simulink model "gm_rmsNormalization"  (R2025a)
settings: Solver=FixedStepDiscrete  StartTime=0.0  StopTime=simStopTime  FixedStep=1  RelTol=1e-3
libraries: simulink x23
(part 1 of 3)
settings Model: Creator=yang  LastModifiedBy=yang
settings OptimizationCC: BlockReduction=off  ConditionallyExecuteInputs=off  DefaultParameterBehavior=Inlined
settings DebuggingCC: InheritedTsInSrcMsg=none  SingleTaskRateTransMsg=error

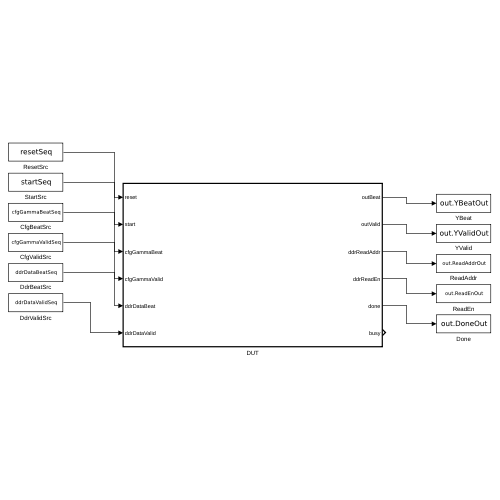
[thumbnail: Simulink's stored preview of the top-level diagram]
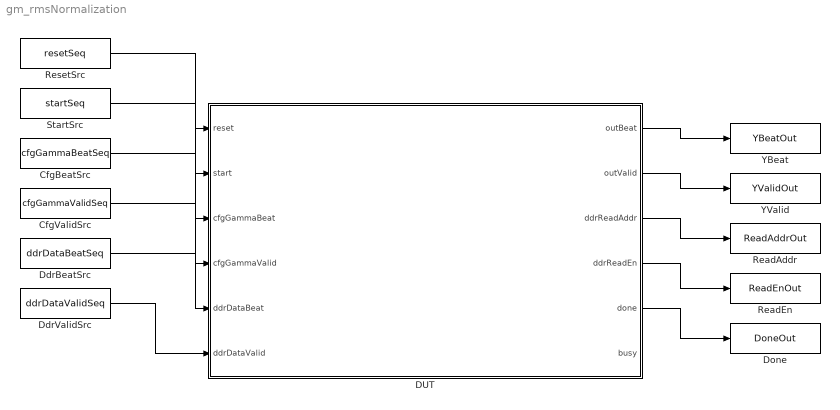
== system gm_rmsNormalization ==
  CfgBeatSrc : FromWorkspace  VariableName=cfgGammaBeatSeq
  CfgValidSrc : FromWorkspace  VariableName=cfgGammaValidSeq
  DUT : Subsystem  TreatAsAtomicUnit=on
  DdrBeatSrc : FromWorkspace  VariableName=ddrDataBeatSeq
  DdrValidSrc : FromWorkspace  VariableName=ddrDataValidSeq
  Done : ToWorkspace  VariableName=DoneOut  SampleTime=-1
  ReadAddr : ToWorkspace  VariableName=ReadAddrOut  SampleTime=-1
  ReadEn : ToWorkspace  VariableName=ReadEnOut  SampleTime=-1
  ResetSrc : FromWorkspace  VariableName=resetSeq
  StartSrc : FromWorkspace  VariableName=startSeq
  YBeat : ToWorkspace  VariableName=YBeatOut  SampleTime=-1
  YValid : ToWorkspace  VariableName=YValidOut  SampleTime=-1
  wires:
  DUT/5(done) -> Done/1
  DUT/4(ddrReadEn) -> ReadEn/1
  DUT/3(ddrReadAddr) -> ReadAddr/1
  DUT/2(outValid) -> YValid/1
  DUT/1(outBeat) -> YBeat/1
  DdrValidSrc/1 -> DUT/6(ddrDataValid)
  DdrBeatSrc/1 -> DUT/5(ddrDataBeat)
  CfgValidSrc/1 -> DUT/4(cfgGammaValid)
  CfgBeatSrc/1 -> DUT/3(cfgGammaBeat)
  StartSrc/1 -> DUT/2(start)
  ResetSrc/1 -> DUT/1(reset)

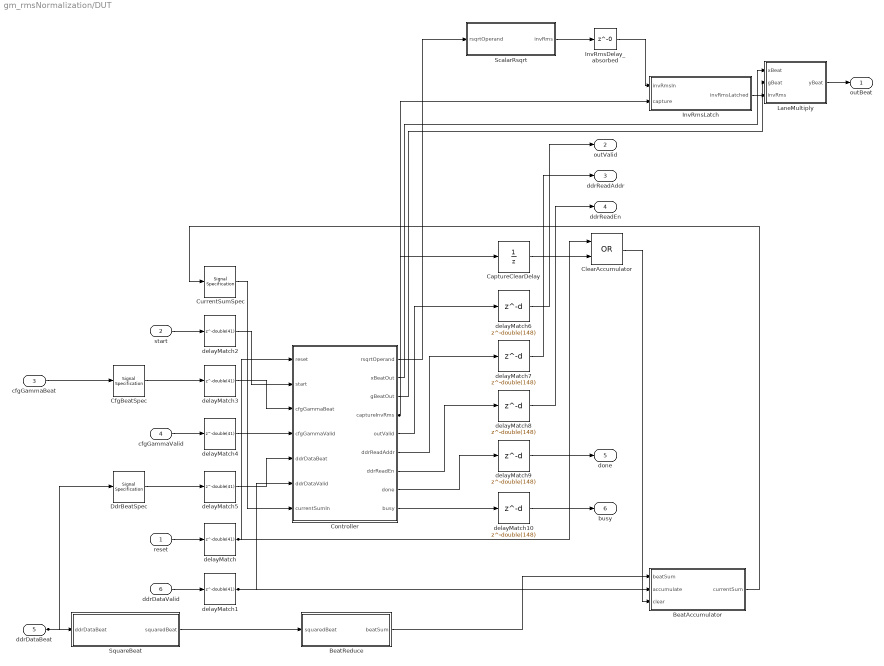
== system gm_rmsNormalization/DUT ==
  reset : Inport  OutDataTypeStr=boolean  PortDimensions=1  SampleTime=1
  start : Inport  Port=2  OutDataTypeStr=boolean  PortDimensions=1  SampleTime=1
  cfgGammaBeat : Inport  Port=3  OutDataTypeStr=single  PortDimensions=[8]  SampleTime=1
  cfgGammaValid : Inport  Port=4  OutDataTypeStr=boolean  PortDimensions=1  SampleTime=1
  ddrDataBeat : Inport  Port=5  OutDataTypeStr=single  PortDimensions=[8]  SampleTime=1
  ddrDataValid : Inport  Port=6  OutDataTypeStr=boolean  PortDimensions=1  SampleTime=1
  BeatAccumulator : Subsystem
  BeatReduce : Subsystem
  CaptureClearDelay : UnitDelay  SampleTime=1
  CfgBeatSpec : SignalSpecification  OutDataTypeStr=single  Dimensions=8
  ClearAccumulator : Logic  Operator=OR  AllPortsSameDT=off  OutDataTypeStr=boolean  SampleTime=1
  Controller : Subsystem
  CurrentSumSpec : SignalSpecification  OutDataTypeStr=single  Dimensions=1
  DdrBeatSpec : SignalSpecification  OutDataTypeStr=single  Dimensions=8
  InvRmsDelay_absorbed : Delay  DelayLength=0
  InvRmsLatch : Subsystem
  LaneMultiply : Subsystem
  ScalarRsqrt : Subsystem
  SquareBeat : Subsystem
  delayMatch{,1..5} (6 alike) : Delay  DelayLength=double(41)  InitialCondition=0  SampleTime=1
  delayMatch{6..10} (5 alike) : Delay  DelayLength=double(148)  InitialCondition=0  SampleTime=1
  outBeat : Outport  SampleTime=1
  outValid : Outport  Port=2  SampleTime=1
  ddrReadAddr : Outport  Port=3  SampleTime=1
  ddrReadEn : Outport  Port=4  SampleTime=1
  done : Outport  Port=5  SampleTime=1
  busy : Outport  Port=6  SampleTime=1
  wires:
  LaneMultiply/1(yBeat) -> outBeat/1
  ClearAccumulator/1 -> BeatAccumulator/3(clear)
  InvRmsDelay_absorbed/1 -> InvRmsLatch/1(invRmsIn)
  delayMatch10/1 -> busy/1
  delayMatch9/1 -> done/1
  delayMatch8/1 -> ddrReadEn/1
  InvRmsLatch/1(invRmsLatched) -> LaneMultiply/3(invRms)
  delayMatch7/1 -> ddrReadAddr/1
  CurrentSumSpec/1 -> Controller/7(currentSumIn)
  delayMatch2/1 -> Controller/2(start)
  ScalarRsqrt/1(invRms) -> InvRmsDelay_absorbed/1
  ddrDataValid/1 -> delayMatch1/1
  DdrBeatSpec/1 -> delayMatch5/1
  cfgGammaValid/1 -> delayMatch4/1
  BeatAccumulator/1(currentSum) -> CurrentSumSpec/1
  CfgBeatSpec/1 -> delayMatch3/1
  Controller/4(captureInvRms) -> CaptureClearDelay/1, InvRmsLatch/2(capture)
  SquareBeat/1(squaredBeat) -> BeatReduce/1(squaredBeat)
  start/1 -> delayMatch2/1
  Controller/7(ddrReadEn) -> delayMatch8/1
  reset/1 -> delayMatch/1
  ddrDataBeat/1 -> SquareBeat/1(ddrDataBeat), DdrBeatSpec/1
  delayMatch5/1 -> Controller/5(ddrDataBeat)
  cfgGammaBeat/1 -> CfgBeatSpec/1
  BeatReduce/1(beatSum) -> BeatAccumulator/1(beatSum)
  delayMatch4/1 -> Controller/4(cfgGammaValid)
  delayMatch/1 -> Controller/1(reset), ClearAccumulator/1
  delayMatch3/1 -> Controller/3(cfgGammaBeat)
  delayMatch1/1 -> Controller/6(ddrDataValid), BeatAccumulator/2(accumulate)
  Controller/5(outValid) -> delayMatch6/1
  Controller/1(rsqrtOperand) -> ScalarRsqrt/1(rsqrtOperand)
  Controller/2(xBeatOut) -> LaneMultiply/1(xBeat)
  Controller/3(gBeatOut) -> LaneMultiply/2(gBeat)
  Controller/6(ddrReadAddr) -> delayMatch7/1
  Controller/8(done) -> delayMatch9/1
  Controller/9(busy) -> delayMatch10/1
  CaptureClearDelay/1 -> ClearAccumulator/2
  delayMatch6/1 -> outValid/1

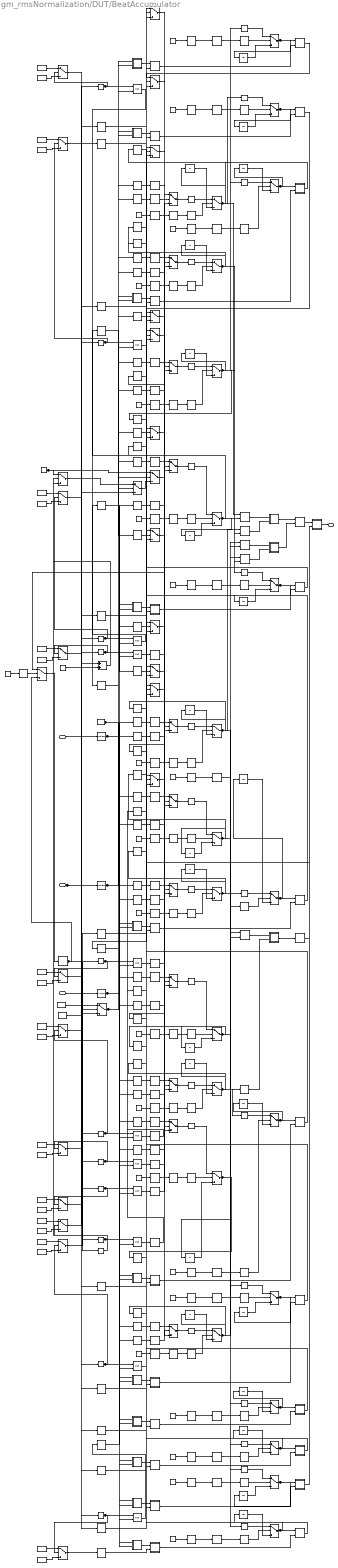
== system gm_rmsNormalization/DUT/BeatAccumulator ==
  beatSum : Inport  OutDataTypeStr=single  PortDimensions=1  SampleTime=1
  accumulate : Inport  Port=2  OutDataTypeStr=boolean  PortDimensions=1  SampleTime=1
  clear : Inport  Port=3  OutDataTypeStr=boolean  PortDimensions=1  SampleTime=1
  AccumulateAdd00 : Subsystem
      mask Display: disp('NFP\nadd');
  AccumulateAdd01 : Subsystem
      mask Display: disp('NFP\nadd');
  AccumulateAdd02 : Subsystem
      mask Display: disp('NFP\nadd');
  AccumulateAdd03 : Subsystem
      mask Display: disp('NFP\nadd');
  AccumulateAdd04 : Subsystem
      mask Display: disp('NFP\nadd');
  AccumulateAdd05 : Subsystem
      mask Display: disp('NFP\nadd');
  AccumulateAdd06 : Subsystem
      mask Display: disp('NFP\nadd');
  AccumulateAdd07 : Subsystem
      mask Display: disp('NFP\nadd');
  AccumulateAdd08 : Subsystem
      mask Display: disp('NFP\nadd');
  AccumulateAdd09 : Subsystem
      mask Display: disp('NFP\nadd');
  AccumulateAdd10 : Subsystem
      mask Display: disp('NFP\nadd');
  AccumulateBool : DataTypeConversion  OutDataTypeStr=boolean
  BankIndexAdd : Sum  OutDataTypeStr=uint8  AccumDataTypeStr=uint8  SampleTime=1
  BankIndexAdvance : Switch  Criteria=u2 ~= 0  Threshold="fi(0,0,1,0,\"hex\",\"0\")"  OutDataTypeStr=uint8  SampleTime=1  SaturateOnIntegerOverflow=off  InputSameDT=off
  BankIndexClear : Switch  Criteria=u2 ~= 0  Threshold="fi(0,0,1,0,\"hex\",\"0\")"  OutDataTypeStr=uint8  SampleTime=1  SaturateOnIntegerOverflow=off  InputSameDT=off
  BankIndexIsLast : simulink/Logic and Bit Operations/Compare To Constant  relop===  const="fi(0,0,8,0,\"hex\",\"0a\")"  OutDataTypeStr=boolean
  BankIndexOne : Constant  OutDataTypeStr=uint8  SampleTime=1
  BankIndexState : Delay  DelayLength=double(1)  InitialCondition=0  SampleTime=1
  BankIndexState_enbsw : Switch  Criteria=u2 ~= 0  Threshold=double(0)  OutDataTypeStr=uint8  SampleTime=1  SaturateOnIntegerOverflow=off  InputSameDT=off
  BankIndexWrap : Switch  Criteria=u2 ~= 0  Threshold="fi(0,0,1,0,\"hex\",\"0\")"  OutDataTypeStr=uint8  SampleTime=1  SaturateOnIntegerOverflow=off  InputSameDT=off
  BankIndexZero : Constant  Value=0  OutDataTypeStr=uint8  SampleTime=1
  BankState00_absorbed : Delay  DelayLength=0
  BankState00_out1bypassMux : Switch  Criteria=u2 ~= 0  Threshold=double(0)  OutDataTypeStr=single  SampleTime=1  SaturateOnIntegerOverflow=off  InputSameDT=off
  BankState01_absorbed : Delay  DelayLength=0
  BankState01_out1bypassMux : Switch  Criteria=u2 ~= 0  Threshold=double(0)  OutDataTypeStr=single  SampleTime=1  SaturateOnIntegerOverflow=off  InputSameDT=off
  BankState02_absorbed : Delay  DelayLength=0
  BankState02_out1bypassMux : Switch  Criteria=u2 ~= 0  Threshold=double(0)  OutDataTypeStr=single  SampleTime=1  SaturateOnIntegerOverflow=off  InputSameDT=off
  BankState03_absorbed : Delay  DelayLength=0
  BankState03_out1bypassMux : Switch  Criteria=u2 ~= 0  Threshold=double(0)  OutDataTypeStr=single  SampleTime=1  SaturateOnIntegerOverflow=off  InputSameDT=off
  BankState04_absorbed : Delay  DelayLength=0
  BankState04_out1bypassMux : Switch  Criteria=u2 ~= 0  Threshold=double(0)  OutDataTypeStr=single  SampleTime=1  SaturateOnIntegerOverflow=off  InputSameDT=off
  BankState05_absorbed : Delay  DelayLength=0
  BankState05_out1bypassMux : Switch  Criteria=u2 ~= 0  Threshold=double(0)  OutDataTypeStr=single  SampleTime=1  SaturateOnIntegerOverflow=off  InputSameDT=off
  BankState06_absorbed : Delay  DelayLength=0
  BankState06_out1bypassMux : Switch  Criteria=u2 ~= 0  Threshold=double(0)  OutDataTypeStr=single  SampleTime=1  SaturateOnIntegerOverflow=off  InputSameDT=off
  BankState07_absorbed : Delay  DelayLength=0
  BankState07_out1bypassMux : Switch  Criteria=u2 ~= 0  Threshold=double(0)  OutDataTypeStr=single  SampleTime=1  SaturateOnIntegerOverflow=off  InputSameDT=off
  BankState08_absorbed : Delay  DelayLength=0
  BankState08_out1bypassMux : Switch  Criteria=u2 ~= 0  Threshold=double(0)  OutDataTypeStr=single  SampleTime=1  SaturateOnIntegerOverflow=off  InputSameDT=off
  BankState09_absorbed : Delay  DelayLength=0
  BankState09_out1bypassMux : Switch  Criteria=u2 ~= 0  Threshold=double(0)  OutDataTypeStr=single  SampleTime=1  SaturateOnIntegerOverflow=off  InputSameDT=off
  BankState10_absorbed : Delay  DelayLength=0
  BankState10_out1bypassMux : Switch  Criteria=u2 ~= 0  Threshold=double(0)  OutDataTypeStr=single  SampleTime=1  SaturateOnIntegerOverflow=off  InputSameDT=off
  BeatSumSingle : DataTypeConversion  OutDataTypeStr=single
  ClearBool : DataTypeConversion  OutDataTypeStr=boolean
  ClearPipe00 : Switch  Criteria=u2 ~= 0  Threshold="fi(0,0,1,0,\"hex\",\"0\")"  OutDataTypeStr=single  SampleTime=1  SaturateOnIntegerOverflow=off  InputSameDT=off
  ClearPipe01 : Switch  Criteria=u2 ~= 0  Threshold="fi(0,0,1,0,\"hex\",\"0\")"  OutDataTypeStr=single  SampleTime=1  SaturateOnIntegerOverflow=off  InputSameDT=off
  ClearPipe02 : Switch  Criteria=u2 ~= 0  Threshold="fi(0,0,1,0,\"hex\",\"0\")"  OutDataTypeStr=single  SampleTime=1  SaturateOnIntegerOverflow=off  InputSameDT=off
  ClearPipe03 : Switch  Criteria=u2 ~= 0  Threshold="fi(0,0,1,0,\"hex\",\"0\")"  OutDataTypeStr=single  SampleTime=1  SaturateOnIntegerOverflow=off  InputSameDT=off
  ClearPipe04 : Switch  Criteria=u2 ~= 0  Threshold="fi(0,0,1,0,\"hex\",\"0\")"  OutDataTypeStr=single  SampleTime=1  SaturateOnIntegerOverflow=off  InputSameDT=off
  ClearPipe05 : Switch  Criteria=u2 ~= 0  Threshold="fi(0,0,1,0,\"hex\",\"0\")"  OutDataTypeStr=single  SampleTime=1  SaturateOnIntegerOverflow=off  InputSameDT=off
  ClearPipe06 : Switch  Criteria=u2 ~= 0  Threshold="fi(0,0,1,0,\"hex\",\"0\")"  OutDataTypeStr=single  SampleTime=1  SaturateOnIntegerOverflow=off  InputSameDT=off
  ClearPipe07 : Switch  Criteria=u2 ~= 0  Threshold="fi(0,0,1,0,\"hex\",\"0\")"  OutDataTypeStr=single  SampleTime=1  SaturateOnIntegerOverflow=off  InputSameDT=off
  ClearPipe08 : Switch  Criteria=u2 ~= 0  Threshold="fi(0,0,1,0,\"hex\",\"0\")"  OutDataTypeStr=single  SampleTime=1  SaturateOnIntegerOverflow=off  InputSameDT=off
  ClearPipe09 : Switch  Criteria=u2 ~= 0  Threshold="fi(0,0,1,0,\"hex\",\"0\")"  OutDataTypeStr=single  SampleTime=1  SaturateOnIntegerOverflow=off  InputSameDT=off
  ClearPipe10 : Switch  Criteria=u2 ~= 0  Threshold="fi(0,0,1,0,\"hex\",\"0\")"  OutDataTypeStr=single  SampleTime=1  SaturateOnIntegerOverflow=off  InputSameDT=off
  FeedbackDelay00_absorbed : Delay  DelayLength=0
  FeedbackDelay00_out1bypassMux : Switch  Criteria=u2 ~= 0  Threshold=double(0)  OutDataTypeStr=single  SampleTime=1  SaturateOnIntegerOverflow=off  InputSameDT=off
  FeedbackDelay01_absorbed : Delay  DelayLength=0
  FeedbackDelay01_out1bypassMux : Switch  Criteria=u2 ~= 0  Threshold=double(0)  OutDataTypeStr=single  SampleTime=1  SaturateOnIntegerOverflow=off  InputSameDT=off
  FeedbackDelay02_absorbed : Delay  DelayLength=0
  FeedbackDelay02_out1bypassMux : Switch  Criteria=u2 ~= 0  Threshold=double(0)  OutDataTypeStr=single  SampleTime=1  SaturateOnIntegerOverflow=off  InputSameDT=off
  FeedbackDelay03_absorbed : Delay  DelayLength=0
  FeedbackDelay03_out1bypassMux : Switch  Criteria=u2 ~= 0  Threshold=double(0)  OutDataTypeStr=single  SampleTime=1  SaturateOnIntegerOverflow=off  InputSameDT=off
  FeedbackDelay04_absorbed : Delay  DelayLength=0
  FeedbackDelay04_out1bypassMux : Switch  Criteria=u2 ~= 0  Threshold=double(0)  OutDataTypeStr=single  SampleTime=1  SaturateOnIntegerOverflow=off  InputSameDT=off
  FeedbackDelay05_absorbed : Delay  DelayLength=0
  FeedbackDelay05_out1bypassMux : Switch  Criteria=u2 ~= 0  Threshold=double(0)  OutDataTypeStr=single  SampleTime=1  SaturateOnIntegerOverflow=off  InputSameDT=off
  FeedbackDelay06_absorbed : Delay  DelayLength=0
  FeedbackDelay06_out1bypassMux : Switch  Criteria=u2 ~= 0  Threshold=double(0)  OutDataTypeStr=single  SampleTime=1  SaturateOnIntegerOverflow=off  InputSameDT=off
  FeedbackDelay07_absorbed : Delay  DelayLength=0
  FeedbackDelay07_out1bypassMux : Switch  Criteria=u2 ~= 0  Threshold=double(0)  OutDataTypeStr=single  SampleTime=1  SaturateOnIntegerOverflow=off  InputSameDT=off
  FeedbackDelay08_absorbed : Delay  DelayLength=0
  FeedbackDelay08_out1bypassMux : Switch  Criteria=u2 ~= 0  Threshold=double(0)  OutDataTypeStr=single  SampleTime=1  SaturateOnIntegerOverflow=off  InputSameDT=off
  FeedbackDelay09_absorbed : Delay  DelayLength=0
  FeedbackDelay09_out1bypassMux : Switch  Criteria=u2 ~= 0  Threshold=double(0)  OutDataTypeStr=single  SampleTime=1  SaturateOnIntegerOverflow=off  InputSameDT=off
  FeedbackDelay10_absorbed : Delay  DelayLength=0
  FeedbackDelay10_out1bypassMux : Switch  Criteria=u2 ~= 0  Threshold=double(0)  OutDataTypeStr=single  SampleTime=1  SaturateOnIntegerOverflow=off  InputSameDT=off
  Gate00 : Subsystem
      mask Display: disp('NFP\nmul');
  Gate001 : Subsystem
      mask Display: disp('NFP\nmul');
  Gate01 : Subsystem
      mask Display: disp('NFP\nmul');
  Gate011 : Subsystem
      mask Display: disp('NFP\nmul');
  Gate02 : Subsystem
      mask Display: disp('NFP\nmul');
  Gate021 : Subsystem
      mask Display: disp('NFP\nmul');
  Gate03 : Subsystem
      mask Display: disp('NFP\nmul');
  Gate031 : Subsystem
      mask Display: disp('NFP\nmul');
  Gate04 : Subsystem
      mask Display: disp('NFP\nmul');
  Gate041 : Subsystem
      mask Display: disp('NFP\nmul');
  Gate05 : Subsystem
      mask Display: disp('NFP\nmul');
  Gate051 : Subsystem
      mask Display: disp('NFP\nmul');
  Gate06 : Subsystem
      mask Display: disp('NFP\nmul');
  Gate061 : Subsystem
      mask Display: disp('NFP\nmul');
  Gate07 : Subsystem
      mask Display: disp('NFP\nmul');
  Gate071 : Subsystem
      mask Display: disp('NFP\nmul');
  Gate08 : Subsystem
      mask Display: disp('NFP\nmul');
  Gate081 : Subsystem
      mask Display: disp('NFP\nmul');
  Gate09 : Subsystem
      mask Display: disp('NFP\nmul');
  Gate091 : Subsystem
      mask Display: disp('NFP\nmul');
  Gate10 : Subsystem
      mask Display: disp('NFP\nmul');
  Gate101 : Subsystem
      mask Display: disp('NFP\nmul');
  HoldOrAcc00 : Switch  Criteria=u2 ~= 0  Threshold="fi(0,0,1,0,\"hex\",\"0\")"  OutDataTypeStr=single  SampleTime=1  SaturateOnIntegerOverflow=off  InputSameDT=off
  HoldOrAcc01 : Switch  Criteria=u2 ~= 0  Threshold="fi(0,0,1,0,\"hex\",\"0\")"  OutDataTypeStr=single  SampleTime=1  SaturateOnIntegerOverflow=off  InputSameDT=off
  HoldOrAcc02 : Switch  Criteria=u2 ~= 0  Threshold="fi(0,0,1,0,\"hex\",\"0\")"  OutDataTypeStr=single  SampleTime=1  SaturateOnIntegerOverflow=off  InputSameDT=off
  HoldOrAcc03 : Switch  Criteria=u2 ~= 0  Threshold="fi(0,0,1,0,\"hex\",\"0\")"  OutDataTypeStr=single  SampleTime=1  SaturateOnIntegerOverflow=off  InputSameDT=off
  HoldOrAcc04 : Switch  Criteria=u2 ~= 0  Threshold="fi(0,0,1,0,\"hex\",\"0\")"  OutDataTypeStr=single  SampleTime=1  SaturateOnIntegerOverflow=off  InputSameDT=off
  HoldOrAcc05 : Switch  Criteria=u2 ~= 0  Threshold="fi(0,0,1,0,\"hex\",\"0\")"  OutDataTypeStr=single  SampleTime=1  SaturateOnIntegerOverflow=off  InputSameDT=off
  HoldOrAcc06 : Switch  Criteria=u2 ~= 0  Threshold="fi(0,0,1,0,\"hex\",\"0\")"  OutDataTypeStr=single  SampleTime=1  SaturateOnIntegerOverflow=off  InputSameDT=off
  HoldOrAcc07 : Switch  Criteria=u2 ~= 0  Threshold="fi(0,0,1,0,\"hex\",\"0\")"  OutDataTypeStr=single  SampleTime=1  SaturateOnIntegerOverflow=off  InputSameDT=off
  HoldOrAcc08 : Switch  Criteria=u2 ~= 0  Threshold="fi(0,0,1,0,\"hex\",\"0\")"  OutDataTypeStr=single  SampleTime=1  SaturateOnIntegerOverflow=off  InputSameDT=off
  HoldOrAcc09 : Switch  Criteria=u2 ~= 0  Threshold="fi(0,0,1,0,\"hex\",\"0\")"  OutDataTypeStr=single  SampleTime=1  SaturateOnIntegerOverflow=off  InputSameDT=off
  HoldOrAcc10 : Switch  Criteria=u2 ~= 0  Threshold="fi(0,0,1,0,\"hex\",\"0\")"  OutDataTypeStr=single  SampleTime=1  SaturateOnIntegerOverflow=off  InputSameDT=off
  Sel00 : simulink/Logic and Bit Operations/Compare To Constant  relop===  const="fi(0,0,8,0,\"hex\",\"00\")"  OutDataTypeStr=boolean
  Sel01 : simulink/Logic and Bit Operations/Compare To Constant  relop===  const="fi(0,0,8,0,\"hex\",\"01\")"  OutDataTypeStr=boolean
  Sel02 : simulink/Logic and Bit Operations/Compare To Constant  relop===  const="fi(0,0,8,0,\"hex\",\"02\")"  OutDataTypeStr=boolean
  Sel03 : simulink/Logic and Bit Operations/Compare To Constant  relop===  const="fi(0,0,8,0,\"hex\",\"03\")"  OutDataTypeStr=boolean
  Sel04 : simulink/Logic and Bit Operations/Compare To Constant  relop===  const="fi(0,0,8,0,\"hex\",\"04\")"  OutDataTypeStr=boolean
  Sel05 : simulink/Logic and Bit Operations/Compare To Constant  relop===  const="fi(0,0,8,0,\"hex\",\"05\")"  OutDataTypeStr=boolean
  Sel06 : simulink/Logic and Bit Operations/Compare To Constant  relop===  const="fi(0,0,8,0,\"hex\",\"06\")"  OutDataTypeStr=boolean
  Sel07 : simulink/Logic and Bit Operations/Compare To Constant  relop===  const="fi(0,0,8,0,\"hex\",\"07\")"  OutDataTypeStr=boolean
  Sel08 : simulink/Logic and Bit Operations/Compare To Constant  relop===  const="fi(0,0,8,0,\"hex\",\"08\")"  OutDataTypeStr=boolean
  Sel09 : simulink/Logic and Bit Operations/Compare To Constant  relop===  const="fi(0,0,8,0,\"hex\",\"09\")"  OutDataTypeStr=boolean
  Sel10 : simulink/Logic and Bit Operations/Compare To Constant  relop===  const="fi(0,0,8,0,\"hex\",\"0a\")"  OutDataTypeStr=boolean
  Sum01 : Subsystem
      mask Display: disp('NFP\nadd');
  Sum0123 : Subsystem
      mask Display: disp('NFP\nadd');
  Sum01234567 : Subsystem
      mask Display: disp('NFP\nadd');
  Sum23 : Subsystem
      mask Display: disp('NFP\nadd');
  Sum45 : Subsystem
      mask Display: disp('NFP\nadd');
  Sum4567 : Subsystem
      mask Display: disp('NFP\nadd');
  Sum67 : Subsystem
      mask Display: disp('NFP\nadd');
  Sum89 : Subsystem
      mask Display: disp('NFP\nadd');
  Sum8910 : Subsystem
      mask Display: disp('NFP\nadd');
  SumAll : Subsystem
      mask Display: disp('NFP\nadd');
  UpdateEn00 : Logic  AllPortsSameDT=off  OutDataTypeStr=boolean  SampleTime=1
  UpdateEn01 : Logic  AllPortsSameDT=off  OutDataTypeStr=boolean  SampleTime=1
  UpdateEn02 : Logic  AllPortsSameDT=off  OutDataTypeStr=boolean  SampleTime=1
  UpdateEn03 : Logic  AllPortsSameDT=off  OutDataTypeStr=boolean  SampleTime=1
  UpdateEn04 : Logic  AllPortsSameDT=off  OutDataTypeStr=boolean  SampleTime=1
  UpdateEn05 : Logic  AllPortsSameDT=off  OutDataTypeStr=boolean  SampleTime=1
  UpdateEn06 : Logic  AllPortsSameDT=off  OutDataTypeStr=boolean  SampleTime=1
  UpdateEn07 : Logic  AllPortsSameDT=off  OutDataTypeStr=boolean  SampleTime=1
  UpdateEn08 : Logic  AllPortsSameDT=off  OutDataTypeStr=boolean  SampleTime=1
  UpdateEn09 : Logic  AllPortsSameDT=off  OutDataTypeStr=boolean  SampleTime=1
  UpdateEn10 : Logic  AllPortsSameDT=off  OutDataTypeStr=boolean  SampleTime=1
  ZeroSingle : Constant  Value=single(0)  OutDataTypeStr=single  SampleTime=1
  delayMatch{,2..4,6,8..10,12,14..16,18,20..22,24,26..28,30,32..34,36,38..40,42,44..46,48,50..52,54,56..58,60,62..64,132..133} (46 alike) : Delay  DelayLength=double(11)  InitialCondition=0  SampleTime=1
  delayMatch{1,7,13,19,25,31,37,43,49,55,61} (11 alike) : Delay  DelayLength=double(1)  InitialCondition=0  SampleTime=1
  delayMatch{66,72..73,79..80,86..87,93..94,100,106} (11 alike) : Delay  DelayLength=double(8)  InitialCondition=0  SampleTime=1
  delayMatch{67..71,74..78,81..85,88..92,95..99,101..105,107..131} (55 alike) : Delay  DelayLength=double(16)  InitialCondition=0  SampleTime=1
  delayMatch{5,11,17,23,29,35,41,47,53,59,65} (11 alike) : Delay  DelayLength=double(10)  InitialCondition=0  SampleTime=1
  delayMatch{134..156} (23 alike) : Delay  DelayLength=double(41)  InitialCondition=0  SampleTime=1
  dtc_const_one{,1..11} (12 alike) : Constant  Value=double(1)  OutDataTypeStr=single  SampleTime=1
  dtc_const_zero{,1..11} (12 alike) : Constant  Value=double(0)  OutDataTypeStr=single  SampleTime=1
  dtc_switch{,1..11} (12 alike) : Switch  Criteria=u2 ~= 0  Threshold=double(0)  OutDataTypeStr=single  SampleTime=1  SaturateOnIntegerOverflow=off  InputSameDT=off
  out0_bypass{,1..21} (22 alike) : UnitDelay  SampleTime=1
  stateControl{,1..22} (23 alike) : Constant  OutDataTypeStr=boolean  SampleTime=1
  currentSum : Outport  SampleTime=1
  wires:
  stateControl7/1 -> delayMatch92/1
  HoldOrAcc00/1 -> ClearPipe00/3
  stateControl12/1 -> delayMatch67/1
  stateControl2/1 -> delayMatch111/1
  delayMatch10/1 -> delayMatch136/1
  UpdateEn02/1 -> delayMatch75/1
  delayMatch83/1 -> delayMatch26/1
  dtc_switch3/1 -> delayMatch73/1
  AccumulateAdd00/1(Out1) -> HoldOrAcc00/1
  ClearPipe08/1 -> BankState08_absorbed/1
  delayMatch106/1 -> Gate101/2(In2)
  dtc_const_zero/1 -> dtc_switch/3
  Sum45/1(Out1) -> Sum4567/1(In1)
  delayMatch18/1 -> HoldOrAcc03/2
  delayMatch63/1 -> ClearPipe10/2
  delayMatch110/1 -> delayMatch9/1
  Gate04/1(Out1) -> Gate041/1(In1)
  out0_bypass5/1 -> FeedbackDelay02_out1bypassMux/3
  dtc_const_one/1 -> dtc_switch/1
  dtc_const_one1/1 -> dtc_switch1/1
  Gate10/1(Out1) -> Gate101/1(In1)
  BankState04_absorbed/1 -> BankState04_out1bypassMux/1
  dtc_const_zero2/1 -> dtc_switch2/3
  dtc_const_zero4/1 -> dtc_switch4/3
  out0_bypass10/1 -> BankState05_out1bypassMux/3
  dtc_const_zero6/1 -> dtc_switch6/3
  UpdateEn03/1 -> delayMatch113/1
  Gate00/1(Out1) -> Gate001/1(In1)
  Gate01/1(Out1) -> Gate011/1(In1)
  Gate08/1(Out1) -> Gate081/1(In1)
  delayMatch116/1 -> delayMatch22/1
  Gate091/1(Out1) -> AccumulateAdd09/2(In2)
  delayMatch76/1 -> delayMatch14/1
  Sum01/1(Out1) -> Sum0123/1(In1)
  delayMatch132/1 -> Sum8910/2(In2)
  Sum01234567/1(Out1) -> SumAll/1(In1)
  Sum23/1(Out1) -> Sum0123/2(In2)
  delayMatch32/1 -> ClearPipe05/1
  BankIndexOne/1 -> BankIndexAdd/2
  dtc_const_one8/1 -> dtc_switch8/1
  stateControl14/1 -> delayMatch74/1
  delayMatch66/1 -> Gate001/2(In2)
  dtc_const_zero5/1 -> dtc_switch5/3
  BankState02_absorbed/1 -> BankState02_out1bypassMux/1
  delayMatch/1 -> HoldOrAcc00/2
  BankIndexClear/1 -> BankIndexState_enbsw/1
  delayMatch126/1 -> delayMatch46/1
  delayMatch143/1 -> BankState08_out1bypassMux/2
  BankIndexState_enbsw/1 -> BankIndexState/1
  accumulate/1 -> dtc_switch/2, AccumulateBool/1
  stateControl9/1 -> delayMatch99/1
  dtc_const_zero9/1 -> dtc_switch9/3
  delayMatch54/1 -> HoldOrAcc09/2
  delayMatch48/1 -> HoldOrAcc08/2
  delayMatch124/1 -> delayMatch44/1
  dtc_switch8/1 -> delayMatch93/1
  out0_bypass2/1 -> BankState01_out1bypassMux/3
  HoldOrAcc09/1 -> ClearPipe09/3
  delayMatch135/1 -> BankState00_out1bypassMux/2
  delayMatch104/1 -> delayMatch57/1
  UpdateEn10/1 -> delayMatch128/1
  delayMatch127/1 -> delayMatch65/1
  delayMatch109/1 -> delayMatch8/1
  delayMatch60/1 -> HoldOrAcc10/2
  stateControl1/1 -> delayMatch71/1
  BankState03_absorbed/1 -> BankState03_out1bypassMux/1
  out0_bypass18/1 -> BankState09_out1bypassMux/3
  delayMatch55/1 -> HoldOrAcc09/3
  delayMatch129/1 -> delayMatch62/1
  delayMatch37/1 -> HoldOrAcc06/3
  HoldOrAcc03/1 -> ClearPipe03/3
  delayMatch130/1 -> delayMatch63/1
  UpdateEn09/1 -> delayMatch102/1
  Sum0123/1(Out1) -> Sum01234567/1(In1)
  stateControl/1 -> delayMatch134/1
  dtc_const_one11/1 -> dtc_switch11/1
  out0_bypass/1 -> BankState00_out1bypassMux/3
  delayMatch30/1 -> HoldOrAcc05/2
  delayMatch53/1 -> delayMatch154/1
  delayMatch85/1 -> delayMatch28/1
  delayMatch57/1 -> ClearPipe09/2
  Sel07/1 -> UpdateEn07/1, dtc_switch8/2
  FeedbackDelay08_out1bypassMux/1 -> AccumulateAdd08/1(In1), out0_bypass17/1
  delayMatch68/1 -> delayMatch/1
  ClearPipe07/1 -> BankState07_absorbed/1
  delayMatch62/1 -> ClearPipe10/1
  delayMatch125/1 -> delayMatch45/1
  ClearBool/1 -> delayMatch104/1, delayMatch110/1, delayMatch98/1, delayMatch91/1, delayMatch84/1, delayMatch77/1, delayMatch115/1, delayMatch125/1, delayMatch120/1, delayMatch130/1, delayMatch70/1, BankIndexClear/2
  stateControl5/1 -> delayMatch85/1
  ClearPipe01/1 -> BankState01_absorbed/1
  delayMatch128/1 -> delayMatch60/1
  FeedbackDelay05_out1bypassMux/1 -> AccumulateAdd05/1(In1), out0_bypass11/1
  FeedbackDelay10_out1bypassMux/1 -> AccumulateAdd10/1(In1), out0_bypass21/1
  stateControl4/1 -> delayMatch116/1
  stateControl21/1 -> delayMatch101/1
  BankState06_out1bypassMux/1 -> out0_bypass12/1, FeedbackDelay06_absorbed/1, delayMatch37/1, Sum67/1(In1)
  delayMatch84/1 -> delayMatch27/1
  out0_bypass13/1 -> FeedbackDelay06_out1bypassMux/3
  delayMatch64/1 -> delayMatch145/1
  delayMatch46/1 -> delayMatch142/1
  stateControl20/1 -> delayMatch95/1
  delayMatch28/1 -> delayMatch139/1
  delayMatch142/1 -> BankState07_out1bypassMux/2
  AccumulateBool/1 -> UpdateEn00/2, BankIndexAdvance/2, UpdateEn10/2, UpdateEn08/2, UpdateEn07/2, UpdateEn05/2, UpdateEn04/2, UpdateEn03/2, UpdateEn02/2, UpdateEn06/2, UpdateEn01/2, UpdateEn09/2
  delayMatch38/1 -> ClearPipe06/1
  BankIndexAdd/1 -> BankIndexWrap/3
  AccumulateAdd08/1(Out1) -> HoldOrAcc08/1
  delayMatch67/1 -> delayMatch5/1
  delayMatch114/1 -> delayMatch20/1
  clear/1 -> ClearBool/1
  BankIndexAdvance/1 -> BankIndexClear/3
  delayMatch19/1 -> HoldOrAcc03/3
  delayMatch88/1 -> delayMatch41/1
  stateControl3/1 -> delayMatch78/1
  delayMatch45/1 -> ClearPipe07/2
  delayMatch4/1 -> delayMatch135/1
  out0_bypass15/1 -> FeedbackDelay07_out1bypassMux/3
  delayMatch147/1 -> FeedbackDelay01_out1bypassMux/2
  UpdateEn01/1 -> delayMatch108/1
  HoldOrAcc01/1 -> ClearPipe01/3
  stateControl17/1 -> delayMatch117/1
  delayMatch36/1 -> HoldOrAcc06/2
  delayMatch9/1 -> ClearPipe01/2
  delayMatch80/1 -> Gate041/2(In2)
  out0_bypass19/1 -> FeedbackDelay09_out1bypassMux/3
  UpdateEn08/1 -> delayMatch96/1
  dtc_const_zero11/1 -> dtc_switch11/3
  dtc_switch5/1 -> delayMatch80/1
  delayMatch97/1 -> delayMatch50/1
  ClearPipe00/1 -> BankState00_absorbed/1
  delayMatch115/1 -> delayMatch21/1
  delayMatch2/1 -> ClearPipe00/1
  dtc_const_zero7/1 -> dtc_switch7/3
  FeedbackDelay04_absorbed/1 -> FeedbackDelay04_out1bypassMux/1
  delayMatch42/1 -> HoldOrAcc07/2
  dtc_switch7/1 -> delayMatch87/1
  ClearPipe10/1 -> BankState10_absorbed/1
  Sum67/1(Out1) -> Sum4567/2(In2)
  out0_bypass1/1 -> FeedbackDelay00_out1bypassMux/3
  delayMatch71/1 -> delayMatch4/1
  dtc_const_one3/1 -> dtc_switch3/1
  stateControl10/1 -> delayMatch105/1
  FeedbackDelay09_absorbed/1 -> FeedbackDelay09_out1bypassMux/1
  Gate011/1(Out1) -> AccumulateAdd01/2(In2)
  delayMatch65/1 -> delayMatch156/1
  HoldOrAcc05/1 -> ClearPipe05/3
  delayMatch90/1 -> delayMatch38/1
  delayMatch8/1 -> ClearPipe01/1
  HoldOrAcc10/1 -> ClearPipe10/3
  stateControl15/1 -> delayMatch112/1
  FeedbackDelay05_absorbed/1 -> FeedbackDelay05_out1bypassMux/1
  delayMatch59/1 -> delayMatch155/1
  delayMatch3/1 -> ClearPipe00/2
  delayMatch139/1 -> BankState04_out1bypassMux/2
  ZeroSingle/1 -> delayMatch129/1, delayMatch124/1, delayMatch109/1, delayMatch103/1, delayMatch114/1, delayMatch90/1, delayMatch97/1, delayMatch69/1, delayMatch83/1, delayMatch76/1, delayMatch119/1
  dtc_const_one5/1 -> dtc_switch5/1
  Sum4567/1(Out1) -> Sum01234567/2(In2)
  delayMatch27/1 -> ClearPipe04/2
  Gate03/1(Out1) -> Gate031/1(In1)
  delayMatch61/1 -> HoldOrAcc10/3
  stateControl18/1 -> delayMatch88/1
  delayMatch137/1 -> BankState02_out1bypassMux/2
  FeedbackDelay09_out1bypassMux/1 -> AccumulateAdd09/1(In1), out0_bypass19/1
  delayMatch153/1 -> FeedbackDelay07_out1bypassMux/2
  delayMatch118/1 -> delayMatch30/1
  dtc_const_one2/1 -> dtc_switch2/1
  Gate02/1(Out1) -> Gate021/1(In1)
  out0_bypass7/1 -> FeedbackDelay03_out1bypassMux/3
  Gate041/1(Out1) -> AccumulateAdd04/2(In2)
  delayMatch24/1 -> HoldOrAcc04/2
  dtc_switch4/1 -> delayMatch79/1
  UpdateEn04/1 -> delayMatch82/1
  delayMatch79/1 -> Gate031/2(In2)
  Sel05/1 -> UpdateEn05/1, dtc_switch6/2
  AccumulateAdd05/1(Out1) -> HoldOrAcc05/1
  BankState02_out1bypassMux/1 -> Sum23/1(In1), FeedbackDelay02_absorbed/1, delayMatch13/1, out0_bypass4/1
  BankIndexWrap/1 -> BankIndexAdvance/1
  delayMatch1/1 -> HoldOrAcc00/3
  delayMatch133/1 -> SumAll/2(In2)
  delayMatch120/1 -> delayMatch33/1
  dtc_switch9/1 -> delayMatch94/1
  AccumulateAdd03/1(Out1) -> HoldOrAcc03/1
  delayMatch151/1 -> FeedbackDelay05_out1bypassMux/2
  delayMatch96/1 -> delayMatch48/1
  delayMatch44/1 -> ClearPipe07/1
  dtc_switch2/1 -> delayMatch72/1
  delayMatch131/1 -> delayMatch64/1
  FeedbackDelay07_out1bypassMux/1 -> AccumulateAdd07/1(In1), out0_bypass15/1
  delayMatch112/1 -> delayMatch23/1
  dtc_switch10/1 -> delayMatch100/1
  delayMatch15/1 -> ClearPipe02/2
  Sel10/1 -> UpdateEn10/1, dtc_switch11/2
  Sel02/1 -> UpdateEn02/1, dtc_switch3/2
  delayMatch14/1 -> ClearPipe02/1
  Sel09/1 -> UpdateEn09/1, dtc_switch10/2
  BankState10_out1bypassMux/1 -> delayMatch132/1, FeedbackDelay10_absorbed/1, out0_bypass20/1, delayMatch61/1
  FeedbackDelay06_out1bypassMux/1 -> AccumulateAdd06/1(In1), out0_bypass13/1
  delayMatch111/1 -> delayMatch10/1
  FeedbackDelay00_out1bypassMux/1 -> AccumulateAdd00/1(In1), out0_bypass1/1
  delayMatch25/1 -> HoldOrAcc04/3
  Sel08/1 -> UpdateEn08/1, dtc_switch9/2
  BankState10_absorbed/1 -> BankState10_out1bypassMux/1
  HoldOrAcc08/1 -> ClearPipe08/3
  Gate051/1(Out1) -> AccumulateAdd05/2(In2)
  Gate001/1(Out1) -> AccumulateAdd00/2(In2)
  delayMatch146/1 -> FeedbackDelay00_out1bypassMux/2
  UpdateEn06/1 -> delayMatch89/1
  AccumulateAdd02/1(Out1) -> HoldOrAcc02/1
  FeedbackDelay03_out1bypassMux/1 -> AccumulateAdd03/1(In1), out0_bypass7/1
  out0_bypass17/1 -> FeedbackDelay08_out1bypassMux/3
  FeedbackDelay02_out1bypassMux/1 -> AccumulateAdd02/1(In1), out0_bypass5/1
  dtc_switch6/1 -> delayMatch86/1
  Sum8910/1(Out1) -> delayMatch133/1
  Sel04/1 -> UpdateEn04/1, dtc_switch5/2
  delayMatch136/1 -> BankState01_out1bypassMux/2
  delayMatch102/1 -> delayMatch54/1
  delayMatch40/1 -> delayMatch141/1
  stateControl8/1 -> delayMatch126/1
  dtc_const_one6/1 -> dtc_switch6/1
  Sel06/1 -> UpdateEn06/1, dtc_switch7/2
  AccumulateAdd01/1(Out1) -> HoldOrAcc01/1
  delayMatch134/1 -> BankIndexState_enbsw/2
  delayMatch49/1 -> HoldOrAcc08/3
  BankState07_out1bypassMux/1 -> FeedbackDelay07_absorbed/1, Sum67/2(In2), delayMatch43/1, out0_bypass14/1
  UpdateEn00/1 -> delayMatch68/1
  dtc_switch1/1 -> delayMatch66/1
  AccumulateAdd07/1(Out1) -> HoldOrAcc07/1
  delayMatch105/1 -> delayMatch58/1
  ClearPipe05/1 -> BankState05_absorbed/1
  dtc_switch/1 -> Gate00/2(In2), Gate10/2(In2), Gate05/2(In2), Gate08/2(In2), Gate06/2(In2), Gate04/2(In2), Gate03/2(In2), Gate09/2(In2), Gate01/2(In2), Gate02/2(In2), Gate07/2(In2)
  delayMatch108/1 -> delayMatch6/1
  delayMatch69/1 -> delayMatch2/1
  BankIndexIsLast/1 -> BankIndexWrap/2
  FeedbackDelay01_absorbed/1 -> FeedbackDelay01_out1bypassMux/1
  BankState04_out1bypassMux/1 -> FeedbackDelay04_absorbed/1, Sum45/1(In1), delayMatch25/1, out0_bypass8/1
  ClearPipe04/1 -> BankState04_absorbed/1
  dtc_switch11/1 -> delayMatch106/1
  BankIndexState/1 -> Sel07/1, Sel04/1, Sel00/1, Sel05/1, Sel09/1, Sel08/1, Sel02/1, Sel06/1, BankIndexIsLast/1, Sel03/1, BankIndexState_enbsw/3, Sel10/1, Sel01/1, BankIndexAdd/1, BankIndexAdvance/3
  BeatSumSingle/1 -> Gate07/1(In1), Gate05/1(In1), Gate02/1(In1), Gate00/1(In1), Gate08/1(In1), Gate06/1(In1), Gate01/1(In1), Gate10/1(In1), Gate04/1(In1), Gate09/1(In1), Gate03/1(In1)
  delayMatch77/1 -> delayMatch15/1
  delayMatch100/1 -> Gate091/2(In2)
  delayMatch113/1 -> delayMatch18/1
  Sum89/1(Out1) -> Sum8910/1(In1)
  stateControl11/1 -> delayMatch131/1
  Gate061/1(Out1) -> AccumulateAdd06/2(In2)
  FeedbackDelay04_out1bypassMux/1 -> AccumulateAdd04/1(In1), out0_bypass9/1
  Gate031/1(Out1) -> AccumulateAdd03/2(In2)
  delayMatch92/1 -> delayMatch40/1
  delayMatch89/1 -> delayMatch36/1
  BankState09_out1bypassMux/1 -> FeedbackDelay09_absorbed/1, Sum89/2(In2), delayMatch55/1, out0_bypass18/1
  Gate07/1(Out1) -> Gate071/1(In1)
  Gate101/1(Out1) -> AccumulateAdd10/2(In2)
  Gate081/1(Out1) -> AccumulateAdd08/2(In2)
  delayMatch33/1 -> ClearPipe05/2
  delayMatch72/1 -> Gate011/2(In2)
  delayMatch150/1 -> FeedbackDelay04_out1bypassMux/2
  delayMatch94/1 -> Gate081/2(In2)
  stateControl6/1 -> delayMatch121/1
  BankState00_absorbed/1 -> BankState00_out1bypassMux/1
  delayMatch75/1 -> delayMatch12/1
  delayMatch21/1 -> ClearPipe03/2
  delayMatch73/1 -> Gate021/2(In2)
  Gate071/1(Out1) -> AccumulateAdd07/2(In2)
  BankIndexZero/1 -> BankIndexWrap/1, BankIndexClear/1
  delayMatch86/1 -> Gate051/2(In2)
  delayMatch119/1 -> delayMatch32/1
  delayMatch98/1 -> delayMatch51/1
  delayMatch82/1 -> delayMatch24/1
  stateControl19/1 -> delayMatch122/1
  BankState01_absorbed/1 -> BankState01_out1bypassMux/1
  Gate05/1(Out1) -> Gate051/1(In1)
  delayMatch99/1 -> delayMatch52/1
  delayMatch156/1 -> FeedbackDelay10_out1bypassMux/2
  delayMatch81/1 -> delayMatch29/1
  delayMatch26/1 -> ClearPipe04/1
  beatSum/1 -> BeatSumSingle/1
  out0_bypass3/1 -> FeedbackDelay01_out1bypassMux/3
  dtc_const_zero8/1 -> dtc_switch8/3
  FeedbackDelay01_out1bypassMux/1 -> AccumulateAdd01/1(In1), out0_bypass3/1
  UpdateEn05/1 -> delayMatch118/1
  BankState07_absorbed/1 -> BankState07_out1bypassMux/1
  delayMatch78/1 -> delayMatch16/1
  delayMatch138/1 -> BankState03_out1bypassMux/2
  HoldOrAcc06/1 -> ClearPipe06/3
  stateControl13/1 -> delayMatch107/1
  AccumulateAdd06/1(Out1) -> HoldOrAcc06/1
  delayMatch34/1 -> delayMatch140/1
  BankState05_absorbed/1 -> BankState05_out1bypassMux/1
  out0_bypass12/1 -> BankState06_out1bypassMux/3
  delayMatch43/1 -> HoldOrAcc07/3
  BankState08_absorbed/1 -> BankState08_out1bypassMux/1
  AccumulateAdd10/1(Out1) -> HoldOrAcc10/1
  delayMatch144/1 -> BankState09_out1bypassMux/2
  delayMatch93/1 -> Gate071/2(In2)
  delayMatch107/1 -> delayMatch11/1
  delayMatch123/1 -> delayMatch42/1
  delayMatch23/1 -> delayMatch149/1
  AccumulateAdd09/1(Out1) -> HoldOrAcc09/1
  FeedbackDelay00_absorbed/1 -> FeedbackDelay00_out1bypassMux/1
  Gate021/1(Out1) -> AccumulateAdd02/2(In2)
  delayMatch50/1 -> ClearPipe08/1
  BankState06_absorbed/1 -> BankState06_out1bypassMux/1
  out0_bypass16/1 -> BankState08_out1bypassMux/3
  out0_bypass21/1 -> FeedbackDelay10_out1bypassMux/3
  delayMatch149/1 -> FeedbackDelay03_out1bypassMux/2
  delayMatch121/1 -> delayMatch34/1
  delayMatch16/1 -> delayMatch137/1
  FeedbackDelay10_absorbed/1 -> FeedbackDelay10_out1bypassMux/1
  BankState08_out1bypassMux/1 -> FeedbackDelay08_absorbed/1, out0_bypass16/1, Sum89/1(In1), delayMatch49/1
  SumAll/1(Out1) -> currentSum/1
  dtc_const_one4/1 -> dtc_switch4/1
  delayMatch17/1 -> delayMatch148/1
  delayMatch51/1 -> ClearPipe08/2
  BankState03_out1bypassMux/1 -> Sum23/2(In2), FeedbackDelay03_absorbed/1, delayMatch19/1, out0_bypass6/1
  delayMatch155/1 -> FeedbackDelay09_out1bypassMux/2
  UpdateEn07/1 -> delayMatch123/1
  delayMatch31/1 -> HoldOrAcc05/3
  out0_bypass14/1 -> BankState07_out1bypassMux/3
  ClearPipe02/1 -> BankState02_absorbed/1
  BankState05_out1bypassMux/1 -> FeedbackDelay05_absorbed/1, Sum45/2(In2), delayMatch31/1, out0_bypass10/1
  HoldOrAcc07/1 -> ClearPipe07/3
  dtc_const_one7/1 -> dtc_switch7/1
  ClearPipe06/1 -> BankState06_absorbed/1
  Sel00/1 -> dtc_switch1/2, UpdateEn00/1
  delayMatch145/1 -> BankState10_out1bypassMux/2
  dtc_const_one10/1 -> dtc_switch10/1
  Sel01/1 -> UpdateEn01/1, dtc_switch2/2
  delayMatch103/1 -> delayMatch56/1
  delayMatch74/1 -> delayMatch17/1
  HoldOrAcc02/1 -> ClearPipe02/3
  FeedbackDelay02_absorbed/1 -> FeedbackDelay02_out1bypassMux/1
  delayMatch117/1 -> delayMatch35/1
  FeedbackDelay03_absorbed/1 -> FeedbackDelay03_out1bypassMux/1
  delayMatch22/1 -> delayMatch138/1
  FeedbackDelay08_absorbed/1 -> FeedbackDelay08_out1bypassMux/1
  FeedbackDelay07_absorbed/1 -> FeedbackDelay07_out1bypassMux/1
  BankState09_absorbed/1 -> BankState09_out1bypassMux/1
  delayMatch95/1 -> delayMatch53/1
  delayMatch5/1 -> delayMatch146/1
  delayMatch39/1 -> ClearPipe06/2
  BankState00_out1bypassMux/1 -> Sum01/1(In1), FeedbackDelay00_absorbed/1, delayMatch1/1, out0_bypass/1
  stateControl16/1 -> delayMatch81/1
  FeedbackDelay06_absorbed/1 -> FeedbackDelay06_out1bypassMux/1
  dtc_const_zero10/1 -> dtc_switch10/3
  Sel03/1 -> dtc_switch4/2, UpdateEn03/1
  AccumulateAdd04/1(Out1) -> HoldOrAcc04/1
  out0_bypass9/1 -> FeedbackDelay04_out1bypassMux/3
  delayMatch56/1 -> ClearPipe09/1
  HoldOrAcc04/1 -> ClearPipe04/3
  delayMatch35/1 -> delayMatch151/1
  delayMatch20/1 -> ClearPipe03/1
  out0_bypass20/1 -> BankState10_out1bypassMux/3
  dtc_const_one9/1 -> dtc_switch9/1
  out0_bypass8/1 -> BankState04_out1bypassMux/3
  BankState01_out1bypassMux/1 -> FeedbackDelay01_absorbed/1, Sum01/2(In2), delayMatch7/1, out0_bypass2/1
  out0_bypass11/1 -> FeedbackDelay05_out1bypassMux/3
  delayMatch140/1 -> BankState05_out1bypassMux/2
  delayMatch70/1 -> delayMatch3/1
  delayMatch13/1 -> HoldOrAcc02/3
  delayMatch91/1 -> delayMatch39/1
  dtc_const_zero3/1 -> dtc_switch3/3
  delayMatch12/1 -> HoldOrAcc02/2
  ClearPipe03/1 -> BankState03_absorbed/1
  Gate09/1(Out1) -> Gate091/1(In1)
  delayMatch122/1 -> delayMatch47/1
  delayMatch141/1 -> BankState06_out1bypassMux/2
  delayMatch47/1 -> delayMatch153/1
  delayMatch41/1 -> delayMatch152/1
  delayMatch11/1 -> delayMatch147/1
  delayMatch101/1 -> delayMatch59/1
  Gate06/1(Out1) -> Gate061/1(In1)
  out0_bypass6/1 -> BankState03_out1bypassMux/3
  delayMatch154/1 -> FeedbackDelay08_out1bypassMux/2
  out0_bypass4/1 -> BankState02_out1bypassMux/3
  delayMatch87/1 -> Gate061/2(In2)
  delayMatch58/1 -> delayMatch144/1
  dtc_const_zero1/1 -> dtc_switch1/3
  delayMatch148/1 -> FeedbackDelay02_out1bypassMux/2
  delayMatch52/1 -> delayMatch143/1
  ClearPipe09/1 -> BankState09_absorbed/1
  delayMatch29/1 -> delayMatch150/1
  stateControl22/1 -> delayMatch127/1
  delayMatch152/1 -> FeedbackDelay06_out1bypassMux/2
  delayMatch6/1 -> HoldOrAcc01/2
  delayMatch7/1 -> HoldOrAcc01/3

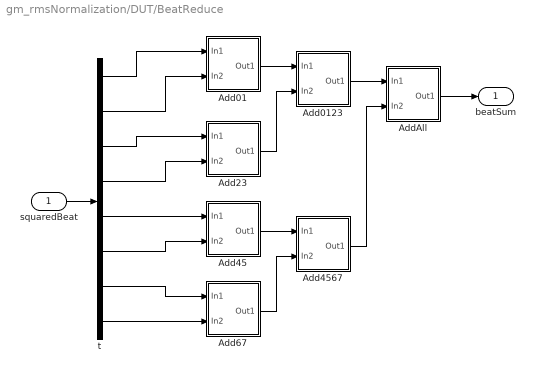
== system gm_rmsNormalization/DUT/BeatReduce ==
  squaredBeat : Inport  OutDataTypeStr=single  PortDimensions=[8]  SampleTime=1
  Add01 : Subsystem
      mask Display: disp('NFP\nadd');
  Add0123 : Subsystem
      mask Display: disp('NFP\nadd');
  Add23 : Subsystem
      mask Display: disp('NFP\nadd');
  Add45 : Subsystem
      mask Display: disp('NFP\nadd');
  Add4567 : Subsystem
      mask Display: disp('NFP\nadd');
  Add67 : Subsystem
      mask Display: disp('NFP\nadd');
  AddAll : Subsystem
      mask Display: disp('NFP\nadd');
  t : Demux  Outputs=8
  beatSum : Outport  SampleTime=1
  wires:
  Add4567/1(Out1) -> AddAll/2(In2)
  Add0123/1(Out1) -> AddAll/1(In1)
  squaredBeat/1 -> t/1
  t/6 -> Add45/2(In2)
  t/1 -> Add01/1(In1)
  t/2 -> Add01/2(In2)
  t/5 -> Add45/1(In1)
  t/3 -> Add23/1(In1)
  AddAll/1(Out1) -> beatSum/1
  t/4 -> Add23/2(In2)
  t/8 -> Add67/2(In2)
  t/7 -> Add67/1(In1)
  Add45/1(Out1) -> Add4567/1(In1)
  Add23/1(Out1) -> Add0123/2(In2)
  Add01/1(Out1) -> Add0123/1(In1)
  Add67/1(Out1) -> Add4567/2(In2)
